simulink model "Exercise9"  (Simulink 7.2)
settings: Solver=ode45  StartTime=0.0  StopTime=1000.0  RelTol=1e-3
undefined symbols (not defined in the file): g, k, M1, M2, mu
settings Model: Creator=Inderjot  LastModifiedBy=Inderjot

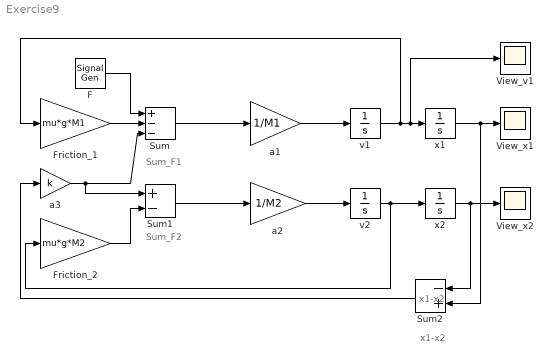
== system Exercise9 ==
  note: Sum_F1
  note: Sum_F2
  note: x1-x2
  note: x1-x2
  F : SignalGenerator  WaveForm=square  Amplitude=-1  Frequency=.001
  Friction_1 : Gain  Gain=mu*g*M1  ParameterDataType=sfix(16)  ParameterScaling=2^0  OutDataType=sfix(16)  OutScaling=2^0
  Friction_2 : Gain  Gain=mu*g*M2  ParameterDataType=sfix(16)  ParameterScaling=2^0  OutDataType=sfix(16)  OutScaling=2^0
  Sum : Sum  Inputs=+--  OutDataType=sfix(16)  OutScaling=2^0
  Sum1 : Sum  Inputs=+-  OutDataType=sfix(16)  OutScaling=2^0
  Sum2 : Sum  Orientation=left  Inputs=-+  OutDataType=sfix(16)  OutScaling=2^0
  View_v1 : Scope
      settings: SaveName=ScopeData2
  View_x1 : Scope
  View_x2 : Scope
      settings: TimeRange=10
  a1 : Gain  Gain=1/M1  ParameterDataType=sfix(16)  ParameterScaling=2^0  OutDataType=sfix(16)  OutScaling=2^0
  a2 : Gain  Gain=1/M2  ParameterDataType=sfix(16)  ParameterScaling=2^0  OutDataType=sfix(16)  OutScaling=2^0
  a3 : Gain  Gain=k  ParameterDataType=sfix(16)  ParameterScaling=2^0  OutDataType=sfix(16)  OutScaling=2^0
  v1 : Integrator
  v2 : Integrator
  x1 : Integrator
  x2 : Integrator
  wires:
  Sum/1 -> a1/1
  Sum1/1 -> a2/1
  a1/1 -> v1/1
  v1/1 -> Friction_1/1, x1/1, View_v1/1
  a2/1 -> v2/1
  v2/1 -> x2/1, Friction_2/1
  x1/1 -> View_x1/1, Sum2/2
  x2/1 -> View_x2/1, Sum2/1
  F/1 -> Sum/1
  Friction_1/1 -> Sum/2
  a3/1 -> Sum/3, Sum1/1
  Sum2/1 -> a3/1
  Friction_2/1 -> Sum1/2
